simulink model "dcmotor_speed_control"  (R2023a)
settings: Solver=FixedStepAuto  StartTime=0.0  StopTime=.5  FixedStep=1e-5  RelTol=1e-3
values from neighbouring files (symbols this model uses):
  B = 0    [parabtl.m]    (also in pmdc_parameter.m; testpara.m)
  J = 0.05    [dcmotor_parameter.m]    (also in parabtl.m; pmdc_parameter.m = 0.00252; testpara.m = 0.00252)
  La = 5.2e-3    (= 0.0052)    [dcmotor_parameter.m]    (also in parabtl.m; pmdc_parameter.m = 0.0017; testpara.m = 0.0017)
  Lf = Laf    (= 0.650632258065)    [dcmotor_parameter.m]
  Ra = 0.32    [dcmotor_parameter.m]    (also in parabtl.m; pmdc_parameter.m = 0.26; testpara.m = 0.26)
  Rf = Uf/If    (= 172.222222222)    [dcmotor_parameter.m]
  Ua = 400    [dcmotor_parameter.m]
  Uf = 310    [dcmotor_parameter.m]
undefined symbols (not defined in the file or in its folder): K
libraries: spsDCVoltageSourceLib x2, spsBreakerLib x1, spsDCMachineLib x1, sps_lib x1
settings Model: Creator=luand  LastModifiedBy=luand
settings SolverCC: ZeroCrossAlgorithm=Adaptive
settings DebuggingCC: IgnoredZcDiagnostic=none

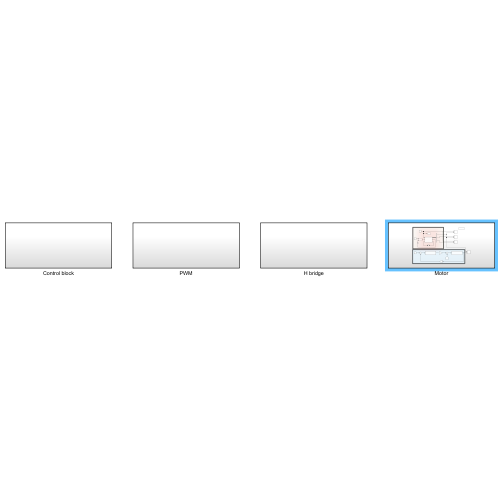
[thumbnail: Simulink's stored preview of the top-level diagram]
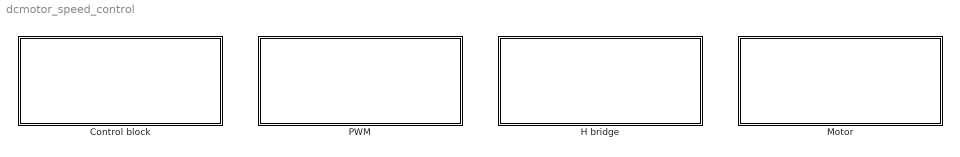
== system dcmotor_speed_control ==
  Control block : Subsystem
  H bridge : Subsystem
  Motor : Subsystem
  PWM : Subsystem

== system dcmotor_speed_control/Control block ==

== system dcmotor_speed_control/H bridge ==

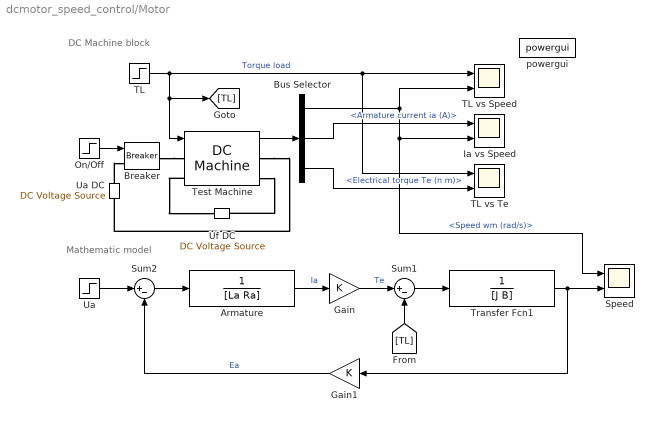
== system dcmotor_speed_control/Motor ==
  note: Mathematic model
  note: DC Machine block
  Armature : TransferFcn  Denominator=[La Ra]
  Breaker : spsBreakerLib/Breaker  InitialState=0  SwitchingTimes="[1/60  5/60]"  External=on  BreakerResistance=0.01  SnubberResistance=1e6  SnubberCapacitance=inf  Measurements=None  MoreParameters=on  NoBreakLoop=off
  Bus Selector : BusSelector  OutputSignals=Speed wm (rad/s),Armature current ia (A),Electrical torque Te (n m)
  Gain : Gain  Gain=K
  Gain1 : Gain  Gain=K
  Ia vs Speed : Scope  NumInputPorts=2
  On/Off : Step  Time=0  SampleTime=0
  Speed : Scope  NumInputPorts=2
  Sum1 : Sum  Inputs=|+-
  Sum2 : Sum  Inputs=|+-
  TL : Step  Time=0.3  After=300  SampleTime=0
  TL vs Speed : Scope  NumInputPorts=2
  TL vs Te : Scope  NumInputPorts=2
  Test Machine : spsDCMachineLib/DC Machine  PresetModel=No  MechanicalLoad=Torque TL  FieldType=Wound  ShowDetailedParameters=on  MeasurementBus=off  RLa=[Ra La]  RLf=[Rf Lf]  Laf=Laf  MachineConstant=Torque constant (N.m/A)  Ke=1.8  Kt=1.8  J=J  Bm=0  Tf=0  w0=0  Ifinit=1.8  TsPowergui=0  TsBlock=-1
  Transfer Fcn1 : TransferFcn  Denominator=[J B]
  Ua : Step  Time=0  After=Ua  SampleTime=0
  Ua DC : spsDCVoltageSourceLib/DC Voltage Source  Amplitude=Ua  Measurements=None
  Uf DC : spsDCVoltageSourceLib/DC Voltage Source  Amplitude=Uf  Measurements=None
  powergui : sps_lib/powergui  Priority=1  SimulationMode=Continuous  SampleTime=50e-6  frequency=60  Iterations=50  frequencyindice=0  Pbase=100e6  ErrMax=1e-4  UnitsV=kV  UnitsW=MW  buscounter=0  FunctionMessages=off  echomessages=off  EnableUseOfTLC=off  CurrentSourceSwitches=off  DisableSnubberDevices=off  DisableRonSwitches=off  DisableVfSwitches=off  DisplayEquations=off  AutomaticDiscreteSolvers=off  SolverType=Tustin/Backward Euler (TBE)  Interpol=off  ExternalGateDelay=off  methode=off  Ts=100  x0status=blocks  SPID=on  SwTol=0  HookPort=off  NonlinearTolerance=1e-4  nMaxIteration=100  ContinueOnMaxIteration=off  RestoreLinks=warning  ResistiveCurrentMeasurement=off  Frange=[0:2:500]  Ylog=off  Xlog=on  ShowGrid=off  save=off  variable=ZData  structure=0  ZoomFFT=off  StartTime=0.0  cycles=1  DisplayStyle=1  fundamental=60  FreqAxis=off  MaxFrequency=1000  frequencyindicesteady=1  RmsSteady=1  display=off
  wires:
  Bus Selector/3 -> TL vs Te/2  "<Electrical torque Te (n m)>"
  Sum2/1 -> Armature/1
  Transfer Fcn1/1 -> Speed/2, Gain1/1
  Ua/1 -> Sum2/1
  Gain/1 -> Sum1/1  "Te"
  On/Off/1 -> Breaker/1
  Gain1/1 -> Sum2/2  "Ea"
  [TL] -> Sum1/2
  Test Machine/1 -> Bus Selector/1
  Sum1/1 -> Transfer Fcn1/1
  Bus Selector/2 -> Ia vs Speed/1  "<Armature current ia (A)>"
  Armature/1 -> Gain/1  "Ia"
  Bus Selector/1 -> TL vs Speed/2, Ia vs Speed/2, Speed/1  "<Speed wm (rad/s)>"
  TL/1 -> Test Machine/1, [TL], TL vs Te/1, TL vs Speed/1  "Torque load"
  connections:
  Ua DC/RConn1 -- Breaker/LConn1
  Test Machine/RConn1 -- Ua DC/LConn1
  Test Machine/RConn2 -- Uf DC/LConn1
  Breaker/RConn1 -- Test Machine/LConn1
  Test Machine/LConn2 -- Uf DC/RConn1

== system dcmotor_speed_control/PWM ==
